simulink model "InvertedPendulTest"  (Simulink 8.3)
settings: Solver=ode45  StartTime=0.0  StopTime=10  RelTol=1e-3
PreLoadFcn:
  | %K=[-1.0000   -2.4146  -34.1064  -10.6737];
values from neighbouring files (symbols this model uses):
  L = 1    [LQRDemo.m]
  m = 0.2    [LQRDemo.m]
  M = 50    [LQRDemo.m]
  X0 = [0,0,0.1,0]    [LQRDemo.m]    (also in MinSearchDemo.m = [20,1,1,0.1,1])
undefined symbols (not defined in the file or in its folder): K
settings Model: Creator=Administrator  LastModifiedBy=李广文
settings OptimizationCC: ExpressionDepthLimit=2147483647
settings DebuggingCC: FcnCallInpInsideContextMsg=UseLocalSettings

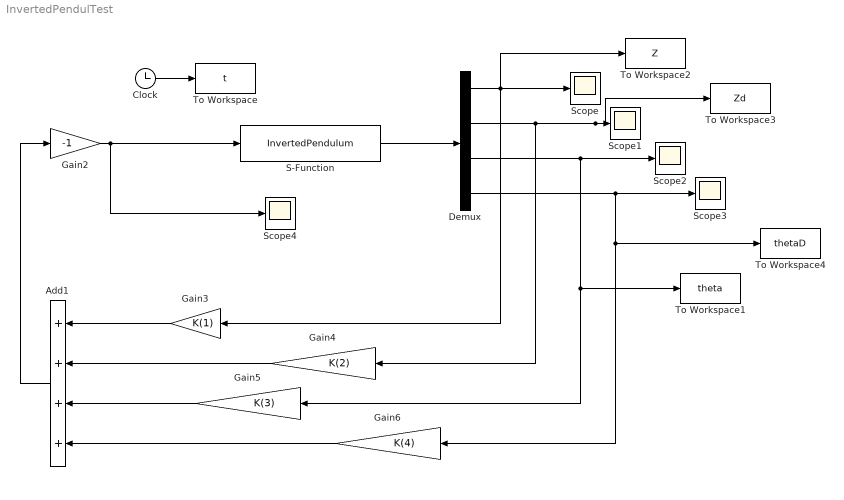
== system InvertedPendulTest ==
  Add1 : Sum  Inputs=++++
  Clock : Clock
  Demux : Demux
  Gain2 : Gain  Gain=-1
  Gain3 : Gain  Gain=K(1)
  Gain4 : Gain  Gain=K(2)
  Gain5 : Gain  Gain=K(3)
  Gain6 : Gain  Gain=K(4)
  S-Function : S-Function  FunctionName=InvertedPendulum  Parameters=L,m,M,X0  EnableBusSupport=off
  Scope{,1..4} (5 alike) : Scope
      Scope2 settings: SaveName=ScopeData2
      Scope3 settings: SaveName=ScopeData3
      Scope4 settings: SaveName=ScopeData4
  To Workspace : ToWorkspace  VariableName=t  SampleTime=-1
  To Workspace1 : ToWorkspace  VariableName=theta  SampleTime=-1
  To Workspace2 : ToWorkspace  VariableName=Z  SampleTime=-1
  To Workspace3 : ToWorkspace  VariableName=Zd  SampleTime=-1
  To Workspace4 : ToWorkspace  VariableName=thetaD  SampleTime=-1
  wires:
  S-Function/1 -> Demux/1
  Demux/1 -> To Workspace2/1, Scope/1, Gain3/1
  Demux/2 -> To Workspace3/1, Scope1/1, Gain4/1
  Demux/3 -> Scope2/1, Gain5/1, To Workspace1/1
  Demux/4 -> Scope3/1, To Workspace4/1, Gain6/1
  Gain3/1 -> Add1/1
  Gain4/1 -> Add1/2
  Gain5/1 -> Add1/3
  Gain6/1 -> Add1/4
  Add1/1 -> Gain2/1
  Gain2/1 -> Scope4/1, S-Function/1
  Clock/1 -> To Workspace/1
